simulink model "Control_DDR_WN"  (R2020a)
settings: Solver=VariableStepAuto  StartTime=0.0  StopTime=inf  RelTol=1e-3
libraries: simulink x3
settings Model: EnablePacing=on  Creator=laptop  LastModifiedBy=laptop

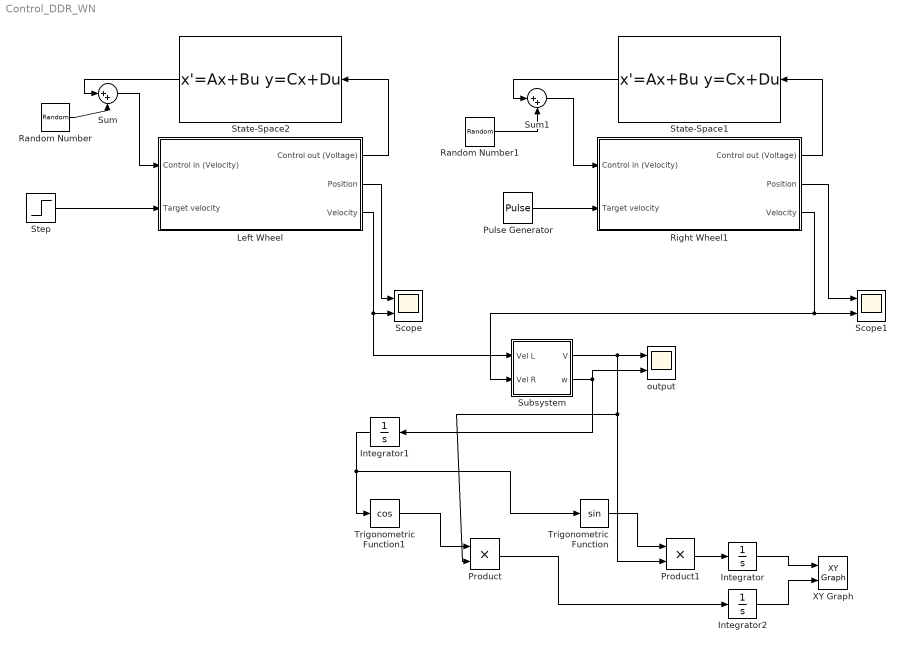
== system Control_DDR_WN ==
  Integrator : Integrator
  Integrator1 : Integrator
  Integrator2 : Integrator
  Left Wheel : Subsystem
  Product : Product
  Product1 : Product
  Pulse Generator : DiscretePulseGenerator  PulseType=Time based  Period=15  PulseWidth=50
  Random Number : RandomNumber  Variance=.001  SampleTime=0.8
  Random Number1 : RandomNumber  Variance=.01  SampleTime=.8
  Right Wheel1 : Subsystem
  Scope : Scope  NumInputPorts=2
  Scope1 : Scope  NumInputPorts=2
  State-Space1 : StateSpace  A=[-0.01099 1.538; -1040 -320]  B=[0.2198; 200]  C=[1 0]  D=0  InitialCondition=0
  State-Space2 : StateSpace  A=[-0.01099 1.538; -1040 -320]  B=[0.2198; 200]  C=[1 0]  D=0  InitialCondition=0
  Step : Step  SampleTime=0
  Subsystem : Subsystem
  Sum : Sum  Inputs=|++
  Sum1 : Sum  Inputs=|++
  Trigonometric Function : Trigonometry
  Trigonometric Function1 : Trigonometry  Operator=cos
  XY Graph : simulink/Sinks/XY Graph  xmin=-10  xmax=10  ymin=-10  ymax=10  st=-1
  output : Scope  NumInputPorts=2
  wires:
  Left Wheel/1(Control out (Voltage)) -> State-Space2/1
  Step/1 -> Left Wheel/2(Target velocity)
  Left Wheel/3(Velocity) -> Subsystem/1(Vel L), Scope/2
  Left Wheel/2(Position) -> Scope/1
  Right Wheel1/1(Control out (Voltage)) -> State-Space1/1
  State-Space1/1 -> Sum1/1
  Pulse Generator/1 -> Right Wheel1/2(Target velocity)
  Right Wheel1/2(Position) -> Scope1/1
  Subsystem/1(V) -> Product1/2, Product/2, output/1
  Subsystem/2(w) -> Integrator1/1, output/2
  Trigonometric Function1/1 -> Product/1
  Right Wheel1/3(Velocity) -> Scope1/2, Subsystem/2(Vel R)
  Product1/1 -> Integrator/1
  Integrator1/1 -> Trigonometric Function/1, Trigonometric Function1/1
  Trigonometric Function/1 -> Product1/1
  Product/1 -> Integrator2/1
  Integrator/1 -> XY Graph/1
  Integrator2/1 -> XY Graph/2
  Random Number/1 -> Sum/2
  Sum/1 -> Left Wheel/1(Control in (Velocity))
  State-Space2/1 -> Sum/1
  Random Number1/1 -> Sum1/2
  Sum1/1 -> Right Wheel1/1(Control in (Velocity))

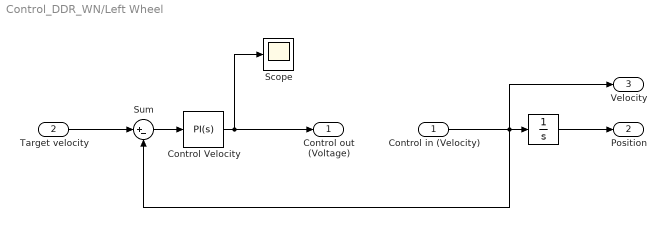
== system Control_DDR_WN/Left Wheel ==
  Control in (Velocity) : Inport
  Target velocity : Inport  Port=2
  " " : Integrator
  Control Velocity : simulink/Continuous/PID Controller  Controller=PI  Form=Parallel  TimeDomain=Continuous-time  UseExternalTs=off  SampleTime=-1  IntegratorMethod=Forward Euler  FilterMethod=Forward Euler  ControllerParametersSource=internal  P=10  I=6  D=0.0632190575311439  UseFilter=on  N=314.98195816595  TunerSelectOption=Transfer Function Based (PID Tuner App)  InitialConditionSource=internal  InitialConditionForIntegrator=0  InitialConditionForFilter=0  DifferentiatorICPrevScaledInput=0  ExternalReset=none  TrackingMode=off  Kt=1  LimitOutput=on  UpperSaturationLimit=12  LowerSaturationLimit=-12  LinearizeAsGain=on  AntiWindupMode=none  Kb=1  POutMin=[]  POutMax=[]  IOutMin=[]  IOutMax=[]  DOutMin=[]  DOutMax=[]  NOutMin=[]  NOutMax=[]  SumOutMin=[]  SumOutMax=[]  SaturationOutMin=[]  SaturationOutMax=[]  PParamMin=[]  PParamMax=[]  IParamMin=[]  IParamMax=[]  DParamMin=[]  DParamMax=[]  NParamMin=[]  NParamMax=[]  KbParamMin=[]  KbParamMax=[]  KtParamMin=[]  KtParamMax=[]  KbOutMin=[]  KbOutMax=[]  KtOutMin=[]  KtOutMax=[]  IntegratorOutMin=[]  IntegratorOutMax=[]  FilterOutMin=[]  FilterOutMax=[]  SumI1OutMin=[]  SumI1OutMax=[]  SumI2OutMin=[]  SumI2OutMax=[]  SumI3OutMin=[]  SumI3OutMax=[]  SumI4OutMin=[]  SumI4OutMax=[]  SumDOutMin=[]  SumDOutMax=[]  DifferentiatorOutMin=[]  DifferentiatorOutMax=[]  FilterDiffOutCoefMin=[]  FilterDiffOutCoefMax=[]  ReciprocalOutMin=[]  ReciprocalOutMax=[]  SumDenOutMin=[]  SumDenOutMax=[]  SumNumOutMin=[]  SumNumOutMax=[]  DivideOutMin=[]  DivideOutMax=[]  UdiffTsProdOutMin=[]  UdiffTsProdOutMax=[]  NTsProdOutMin=[]  NTsProdOutMax=[]  UintegralTsProdOutMin=[]  UintegralTsProdOutMax=[]  UngainTsProdOutMin=[]  UngainTsProdOutMax=[]  IntegratorContinuousStateAttributes=''  IntegratorStateMustResolveToSignalObject=off  IntegratorRTWStateStorageClass=Auto  FilterContinuousStateAttributes=''  FilterStateMustResolveToSignalObject=off  FilterRTWStateStorageClass=Auto  ParallelPVariant=InternalParameters  IdealPVariant=Disabled  IVariant=InternalParameters  DVariant=Disabled  IntegratorVariant=Continuous  SatVariant=Enabled  AWVariant=Passthrough  PCopyVariant=Disabled  TRVariant=Disabled  FdbkBlocksVariant=Forward  IdealPFdbkVariant=Disabled  SatFdbkVariant=Disabled  DerivativeFilterVariant=Disabled  NVariant=Disabled  NCopyVariant=Disabled_SignalSpec  FilterICVariant=Disabled  IntegratorICVariant=InternalICs  ExternalResetVariant=Disabled  TRSumVariant=Passthrough  SumFdbkVariant=Disabled  SumVariant=Sum_PI  TsampFilterVariant=InternalTs  TsampNgainVariant=Passthrough  TsampIntegralVariant=Passthrough
  Scope : Scope
  Sum : Sum  Inputs=|+-
  Control out (Voltage) : Outport
  Position : Outport  Port=2
  Velocity : Outport  Port=3
  wires:
  Control Velocity/1 -> Control out (Voltage)/1, Scope/1
  Control in (Velocity)/1 -> " "/1, Sum/2, Velocity/1
  Target velocity/1 -> Sum/1
  " "/1 -> Position/1
  Sum/1 -> Control Velocity/1

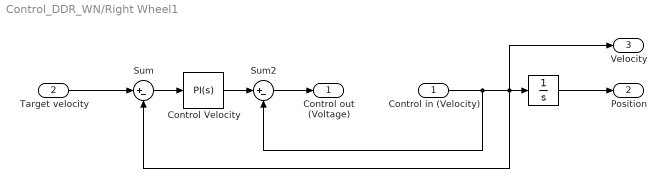
== system Control_DDR_WN/Right Wheel1 ==
  Control in (Velocity) : Inport
  Target velocity : Inport  Port=2
  " " : Integrator
  Control Velocity : simulink/Continuous/PID Controller  Controller=PI  Form=Parallel  TimeDomain=Continuous-time  UseExternalTs=off  SampleTime=-1  IntegratorMethod=Forward Euler  FilterMethod=Forward Euler  ControllerParametersSource=internal  P=10  I=6  D=0.0632190575311439  UseFilter=on  N=314.98195816595  TunerSelectOption=Transfer Function Based (PID Tuner App)  InitialConditionSource=internal  InitialConditionForIntegrator=0  InitialConditionForFilter=0  DifferentiatorICPrevScaledInput=0  ExternalReset=none  TrackingMode=off  Kt=1  LimitOutput=on  UpperSaturationLimit=12  LowerSaturationLimit=-12  LinearizeAsGain=on  AntiWindupMode=none  Kb=1  POutMin=[]  POutMax=[]  IOutMin=[]  IOutMax=[]  DOutMin=[]  DOutMax=[]  NOutMin=[]  NOutMax=[]  SumOutMin=[]  SumOutMax=[]  SaturationOutMin=[]  SaturationOutMax=[]  PParamMin=[]  PParamMax=[]  IParamMin=[]  IParamMax=[]  DParamMin=[]  DParamMax=[]  NParamMin=[]  NParamMax=[]  KbParamMin=[]  KbParamMax=[]  KtParamMin=[]  KtParamMax=[]  KbOutMin=[]  KbOutMax=[]  KtOutMin=[]  KtOutMax=[]  IntegratorOutMin=[]  IntegratorOutMax=[]  FilterOutMin=[]  FilterOutMax=[]  SumI1OutMin=[]  SumI1OutMax=[]  SumI2OutMin=[]  SumI2OutMax=[]  SumI3OutMin=[]  SumI3OutMax=[]  SumI4OutMin=[]  SumI4OutMax=[]  SumDOutMin=[]  SumDOutMax=[]  DifferentiatorOutMin=[]  DifferentiatorOutMax=[]  FilterDiffOutCoefMin=[]  FilterDiffOutCoefMax=[]  ReciprocalOutMin=[]  ReciprocalOutMax=[]  SumDenOutMin=[]  SumDenOutMax=[]  SumNumOutMin=[]  SumNumOutMax=[]  DivideOutMin=[]  DivideOutMax=[]  UdiffTsProdOutMin=[]  UdiffTsProdOutMax=[]  NTsProdOutMin=[]  NTsProdOutMax=[]  UintegralTsProdOutMin=[]  UintegralTsProdOutMax=[]  UngainTsProdOutMin=[]  UngainTsProdOutMax=[]  IntegratorContinuousStateAttributes=''  IntegratorStateMustResolveToSignalObject=off  IntegratorRTWStateStorageClass=Auto  FilterContinuousStateAttributes=''  FilterStateMustResolveToSignalObject=off  FilterRTWStateStorageClass=Auto  ParallelPVariant=InternalParameters  IdealPVariant=Disabled  IVariant=InternalParameters  DVariant=Disabled  IntegratorVariant=Continuous  SatVariant=Enabled  AWVariant=Passthrough  PCopyVariant=Disabled  TRVariant=Disabled  FdbkBlocksVariant=Forward  IdealPFdbkVariant=Disabled  SatFdbkVariant=Disabled  DerivativeFilterVariant=Disabled  NVariant=Disabled  NCopyVariant=Disabled_SignalSpec  FilterICVariant=Disabled  IntegratorICVariant=InternalICs  ExternalResetVariant=Disabled  TRSumVariant=Passthrough  SumFdbkVariant=Disabled  SumVariant=Sum_PI  TsampFilterVariant=InternalTs  TsampNgainVariant=Passthrough  TsampIntegralVariant=Passthrough
  Sum : Sum  Inputs=|+-
  Sum2 : Sum  Inputs=|+-
  Control out (Voltage) : Outport
  Position : Outport  Port=2
  Velocity : Outport  Port=3
  wires:
  Sum/1 -> Control Velocity/1
  " "/1 -> Position/1
  Target velocity/1 -> Sum/1
  Control in (Velocity)/1 -> Velocity/1, Sum/2, " "/1, Sum2/2
  Sum2/1 -> Control out (Voltage)/1
  Control Velocity/1 -> Sum2/1

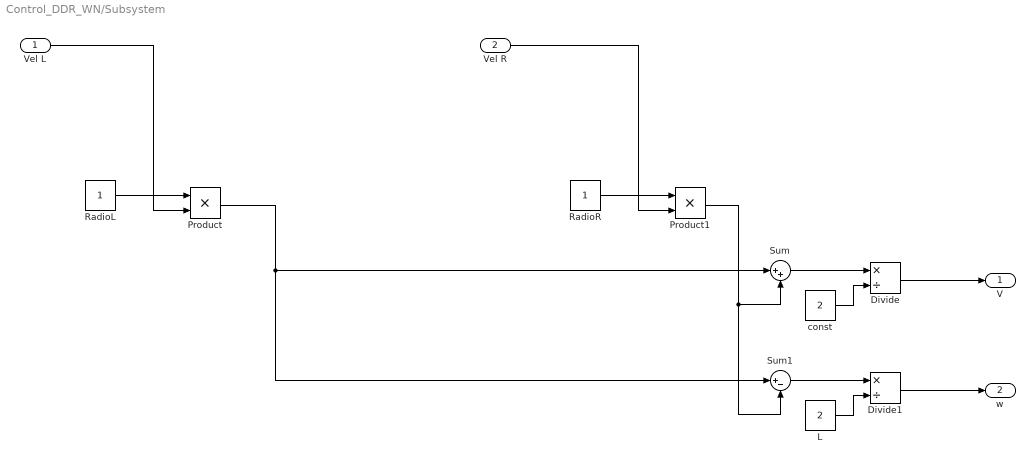
== system Control_DDR_WN/Subsystem ==
  Vel L : Inport
  Vel R : Inport  Port=2
  Divide : Product  Inputs=*/
  Divide1 : Product  Inputs=*/
  L : Constant  Value=2
  Product : Product
  Product1 : Product
  RadioL : Constant
  RadioR : Constant
  Sum : Sum  Inputs=|++
  Sum1 : Sum  Inputs=|+-
  const : Constant  Value=2
  V : Outport
  w : Outport  Port=2
  wires:
  RadioL/1 -> Product/1
  Sum1/1 -> Divide1/1
  Product1/1 -> Sum1/2, Sum/2
  L/1 -> Divide1/2
  Vel L/1 -> Product/2
  const/1 -> Divide/2
  Product/1 -> Sum1/1, Sum/1
  RadioR/1 -> Product1/1
  Sum/1 -> Divide/1
  Vel R/1 -> Product1/2
  Divide/1 -> V/1
  Divide1/1 -> w/1
